simulink model "visual_servoing_control"  (R2020a)
settings: Solver=FixedStepAuto  StartTime=0.0  StopTime=inf  RelTol=1e-3
model workspace (MAT data in the model file):
  SL_ROS_VariableLengthArrays_MaxSizes.CommonInfo.ArrayTruncateAction = 'EmitWarning'
  SL_ROS_VariableLengthArrays_MaxSizes.MsgTypeMap = containers.Map
  SL_ROS_VariableLengthArrays_MaxSizes.MsgTypeMap.serialization.keys = {'sensor_msgs/Image'}
  SL_ROS_VariableLengthArrays_MaxSizes.MsgTypeMap.serialization.values{1}(1).PropertyName = 'Data'
  SL_ROS_VariableLengthArrays_MaxSizes.MsgTypeMap.serialization.values{1}(1).DataType = 'uint8'
  SL_ROS_VariableLengthArrays_MaxSizes.MsgTypeMap.serialization.values{1}(1).MaxLength = 921600
  SL_ROS_VariableLengthArrays_MaxSizes.MsgTypeMap.serialization.values{1}(2).PropertyName = 'Encoding'
  SL_ROS_VariableLengthArrays_MaxSizes.MsgTypeMap.serialization.values{1}(2).DataType = 'uint8'
  SL_ROS_VariableLengthArrays_MaxSizes.MsgTypeMap.serialization.values{1}(2).MaxLength = 128
  SL_ROS_VariableLengthArrays_MaxSizes.MsgTypeMap.serialization.uniformity = 0
  SL_ROS_VariableLengthArrays_MaxSizes.MsgTypeMap.serialization.keyType = 'char'
  SL_ROS_VariableLengthArrays_MaxSizes.MsgTypeMap.serialization.valueType = 'any'
undefined symbols (not defined in the file or in its folder): DiscIntNeverNeededParam
libraries: robotlib x16, robotmaniplib x1
settings Model: Creator=Vuong  LastModifiedBy=Vuong
settings OptimizationCC: EnhancedBackFolding=on  PassReuseOutputArgsAs=Individual arguments  ZeroExternalMemoryAtStartup=off  ZeroInternalMemoryAtStartup=off  MaxStackSize=64  OptimizeBlockOrder=speed  DifferentSizesBufferReuse=on  OptimizationCustomize=off  EfficientTunableParamExpr=on
settings DebuggingCC: ParameterTunabilityLossMsg=error
settings HardwareCC: ProdBitPerPointer=32  ProdBitPerSizeT=32  ProdBitPerPtrDiffT=32  ProdLargestAtomicFloat=None  ProdIntDivRoundTo=Undefined  ProdEndianess=Unspecified  ProdWordSize=32  ProdHWDeviceType=Generic->Unspecified (assume 32-bit Generic)  UseEmbeddedCoderFeatures=off
settings SFSimCC: MATLABDynamicMemAlloc=off
settings RTWCC: SystemTargetFile=ert.tlc  HardwareBoard=Robot Operating System (ROS)  TemplateMakefile=ert_default_tmf  Toolchain=Catkin  TargetLang=C++
settings CodeAppCC: ForceParamTrailComments=on  IgnoreCustomStorageClasses=off  OperatorAnnotations=on  SimulinkDataObjDesc=on  SFDataObjDesc=on  InsertBlockDesc=on
settings ERTTargetCC: SupportNonInlinedSFcns=on

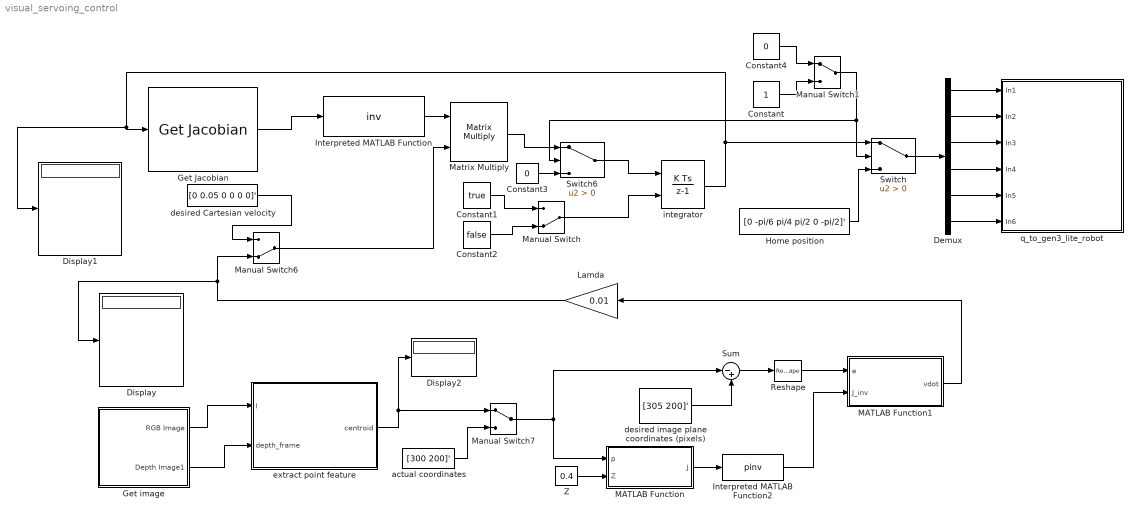
== system visual_servoing_control ==
  Constant : Constant
  Constant1 : Constant  Value=true
  Constant2 : Constant  Value=false
  Constant3 : Constant  Value=0
  Constant4 : Constant  Value=0
  Demux : Demux  Outputs=6
  Display : Display
  Display1 : Display
  Display2 : Display
  Get Jacobian : robotmaniplib/Get Jacobian  RigidBodyTree=gen3_lite_robot  EndEffector=END_EFFECTOR  SimulateUsing=Interpreted execution
      settings: SourceProductBaseCode=RO
  Get image : Subsystem
  Home position : Constant  Value=[0 -pi/6 pi/4 pi/2 0 -pi/2]'
  Interpreted MATLAB Function : MATLABFcn  MATLABFcn=inv  Output1D=off
  Interpreted MATLAB Function2 : MATLABFcn  MATLABFcn=pinv  Output1D=off
  Lamda : Gain  Gain=0.01
  MATLAB Function : MATLAB Function  TreatAsAtomicUnit=on
  MATLAB Function1 : MATLAB Function  TreatAsAtomicUnit=on
  Manual Switch : ManualSwitch  CurrentSetting=0
  Manual Switch1 : ManualSwitch
  Manual Switch6 : ManualSwitch  CurrentSetting=0
  Manual Switch7 : ManualSwitch
  Matrix Multiply : Product  Multiplication=Matrix(*)
  Reshape : Reshape
  Sum : Sum  Inputs=|-+
  Switch : Switch  Criteria=u2 > Threshold
  Switch6 : Switch  Criteria=u2 > Threshold
  Z : Constant  Value=0.4
  actual coordinates : Constant  Value=[300 200]'  VectorParams1D=off
  desired Cartesian velocity : Constant  Value=[0 0.05 0 0 0 0]'
  desired image plane coordinates (pixels) : Constant  Value=[305 200]'  VectorParams1D=off
  extract point feature : MATLAB Function  TreatAsAtomicUnit=on
  integrator : DiscreteIntegrator  ExternalReset=level  SampleTime=-1  LimitOutput=on  UpperSaturationLimit=pi  LowerSaturationLimit=-pi  ICPrevOutput=DiscIntNeverNeededParam  ICPrevScaledInput=DiscIntNeverNeededParam
  q_to_gen3_lite_robot : Subsystem
  wires:
  integrator/1 -> Get Jacobian/1, Display1/1, Switch/1
  desired Cartesian velocity/1 -> Manual Switch6/1
  Get Jacobian/1 -> Interpreted MATLAB Function/1
  Interpreted MATLAB Function/1 -> Matrix Multiply/1
  desired image plane coordinates (pixels)/1 -> Sum/2
  MATLAB Function/1(J) -> Interpreted MATLAB Function2/1
  Interpreted MATLAB Function2/1 -> MATLAB Function1/2(J_inv)
  Lamda/1 -> Manual Switch6/2, Display/1
  Manual Switch6/1 -> Matrix Multiply/2
  Z/1 -> MATLAB Function/2(Z)
  Sum/1 -> Reshape/1
  Reshape/1 -> MATLAB Function1/1(e)
  MATLAB Function1/1(vdot) -> Lamda/1
  Manual Switch7/1 -> Sum/1, MATLAB Function/1(p)
  actual coordinates/1 -> Manual Switch7/2
  extract point feature/1(centroid) -> Display2/1, Manual Switch7/1
  Get image/1(RGB Image) -> extract point feature/1(I)
  Get image/2(Depth Image1) -> extract point feature/2(depth_frame)
  Demux/1 -> q_to_gen3_lite_robot/1(In1)
  Demux/2 -> q_to_gen3_lite_robot/2(In2)
  Demux/3 -> q_to_gen3_lite_robot/3(In3)
  Demux/4 -> q_to_gen3_lite_robot/4(In4)
  Demux/5 -> q_to_gen3_lite_robot/5(In5)
  Demux/6 -> q_to_gen3_lite_robot/6(In6)
  Constant1/1 -> Manual Switch/1
  Constant2/1 -> Manual Switch/2
  Manual Switch/1 -> integrator/2
  Matrix Multiply/1 -> Switch6/1
  Switch6/1 -> integrator/1
  Constant3/1 -> Switch6/3
  Switch/1 -> Demux/1
  Home position/1 -> Switch/3
  Constant4/1 -> Manual Switch1/1
  Constant/1 -> Manual Switch1/2
  Manual Switch1/1 -> Switch6/2, Switch/2

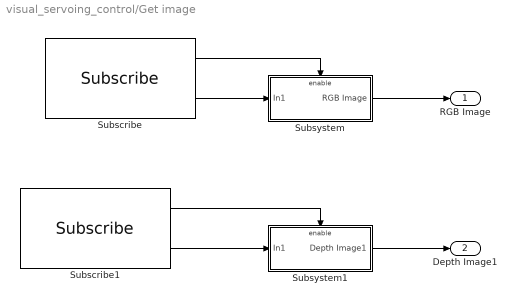
== system visual_servoing_control/Get image ==
  Subscribe : robotlib/Subscribe  topicSource=Select from ROS network  topic=/r200/camera/color/image_raw  messageType=sensor_msgs/Image  sampleTime=-1  messageQueueLength=1
  Subscribe1 : robotlib/Subscribe  topicSource=Select from ROS network  topic=/r200/camera/depth/image_raw  messageType=sensor_msgs/Image  sampleTime=-1  messageQueueLength=1
  Subsystem : Subsystem
  Subsystem1 : Subsystem
  RGB Image : Outport
  Depth Image1 : Outport  Port=2
  wires:
  Subscribe/1 -> Subsystem/Enable
  Subscribe1/1 -> Subsystem1/Enable
  Subsystem/1(RGB Image) -> RGB Image/1
  Subsystem1/1(Depth Image1) -> Depth Image1/1
  Subscribe/2 -> Subsystem/1(In1)
  Subscribe1/2 -> Subsystem1/1(In1)

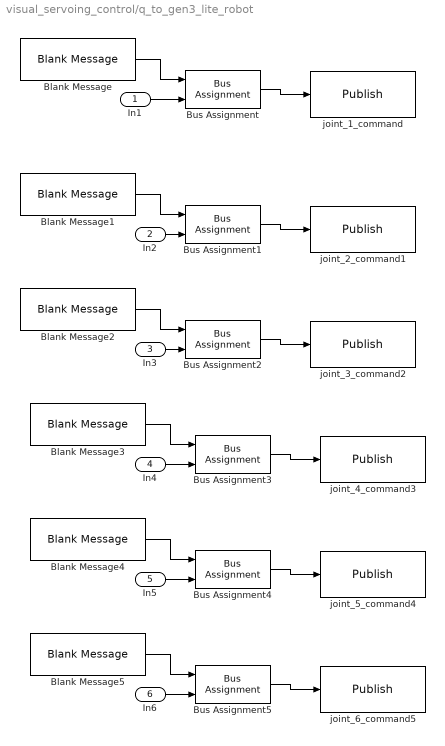
== system visual_servoing_control/q_to_gen3_lite_robot ==
  In1 : Inport
  In2 : Inport  Port=2
  In3 : Inport  Port=3
  In4 : Inport  Port=4
  In5 : Inport  Port=5
  In6 : Inport  Port=6
  Blank Message{,1..5} (6 alike) : robotlib/Blank Message  messageClass=Message  entityType=std_msgs/Float64  messageType=std_msgs/Float64  SampleTime=inf
  Bus Assignment{,1..5} (6 alike) : BusAssignment  AssignedSignals=Data
  joint_1_command : robotlib/Publish  topicSource=Select from ROS network  topic=/my_gen3_lite/joint_1_position_controller/command  messageType=std_msgs/Float64  messageQueueLength=1
  joint_2_command1 : robotlib/Publish  topicSource=Select from ROS network  topic=/my_gen3_lite/joint_2_position_controller/command  messageType=std_msgs/Float64  messageQueueLength=1
  joint_3_command2 : robotlib/Publish  topicSource=Select from ROS network  topic=/my_gen3_lite/joint_3_position_controller/command  messageType=std_msgs/Float64  messageQueueLength=1
  joint_4_command3 : robotlib/Publish  topicSource=Select from ROS network  topic=/my_gen3_lite/joint_4_position_controller/command  messageType=std_msgs/Float64  messageQueueLength=1
  joint_5_command4 : robotlib/Publish  topicSource=Select from ROS network  topic=/my_gen3_lite/joint_5_position_controller/command  messageType=std_msgs/Float64  messageQueueLength=1
  joint_6_command5 : robotlib/Publish  topicSource=Select from ROS network  topic=/my_gen3_lite/joint_6_position_controller/command  messageType=std_msgs/Float64  messageQueueLength=1
  wires:
  Bus Assignment2/1 -> joint_3_command2/1
  Bus Assignment5/1 -> joint_6_command5/1
  Blank Message5/1 -> Bus Assignment5/1
  Bus Assignment1/1 -> joint_2_command1/1
  Blank Message1/1 -> Bus Assignment1/1
  Blank Message4/1 -> Bus Assignment4/1
  Bus Assignment4/1 -> joint_5_command4/1
  Blank Message3/1 -> Bus Assignment3/1
  Bus Assignment/1 -> joint_1_command/1
  Blank Message/1 -> Bus Assignment/1
  Blank Message2/1 -> Bus Assignment2/1
  Bus Assignment3/1 -> joint_4_command3/1
  In1/1 -> Bus Assignment/2
  In2/1 -> Bus Assignment1/2
  In3/1 -> Bus Assignment2/2
  In4/1 -> Bus Assignment3/2
  In5/1 -> Bus Assignment4/2
  In6/1 -> Bus Assignment5/2

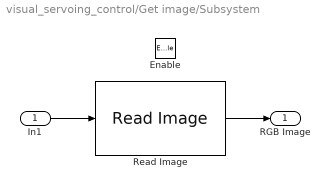
== system visual_servoing_control/Get image/Subsystem ==
  In1 : Inport
  Enable : EnablePort
  Read Image : robotlib/Read Image  MaximumImageSize=[480, 640]  ImageEncoding=rgb8  ShowAlphaOutput=off  ShowErrorCodeOutput=off  VariableSizeOutputs=off
      settings: SourceProductBaseCode=RR
  RGB Image : Outport
  wires:
  Read Image/1 -> RGB Image/1
  In1/1 -> Read Image/1

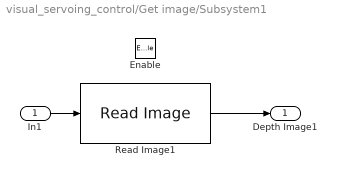
== system visual_servoing_control/Get image/Subsystem1 ==
  In1 : Inport
  Enable : EnablePort
  Read Image1 : robotlib/Read Image  MaximumImageSize=[480, 640]  ImageEncoding=16uc1  ShowAlphaOutput=off  ShowErrorCodeOutput=off  VariableSizeOutputs=off
      settings: SourceProductBaseCode=RR
  Depth Image1 : Outport
  wires:
  In1/1 -> Read Image1/1
  Read Image1/1 -> Depth Image1/1

== matlab function visual_servoing_control/MATLAB Function1 ==
  data: e input; vdot output; J_inv input
function vdot = multiply(e,J_inv)
vdot = J_inv*e;

== matlab function visual_servoing_control/MATLAB Function ==
  data: p input; J output; Z input
function J = visual_jacobian(p,Z)
%test point
%m(u,v) is coordinate of image point (Matlab coordinate relative to
%top-left point
u = p(1,1);
v = p(2,1);
img_size = [480;640];
%img_size = [1280;1024];
%p is pixel coordinate p =[u_hat;v_hat] relative to principle point[u0;v0]

%pixel size
rho = 1e-06;
%focal length
f = 0.008;
%principle point
u0 = img_size(1,1)/2;
v0 = img_size(2,1)/2;
u_hat = u - u0;
v_hat = v - v0;
f = f/rho;
%f = 800;
J = [-f/Z 0 u_hat/Z u_hat*v_hat/f -(f^2+u_hat^2)/f v_hat;
    0 -f/Z v_hat/Z (f^2+v_hat^2)/f -(u_hat*v_hat)/f -u_hat];

== matlab function visual_servoing_control/extract point feature ==
  data: I input; centroid output; depth_frame input
function centroid = extract_feature(I, depth_frame)
    centroid =zeros(2,1);
    coder.extrinsic('segment_extrinsic');
    centroid = segment_extrinsic(I, depth_frame);
